simulink model "charttest"  (R2014b)
settings: Solver=ode45  StartTime=0.0  StopTime=30  RelTol=1e-3
libraries: simulink x2
settings Model: Creator=Edoardo  LastModifiedBy=Edoardo
settings SolverCC: PositivePriorityOrder=on

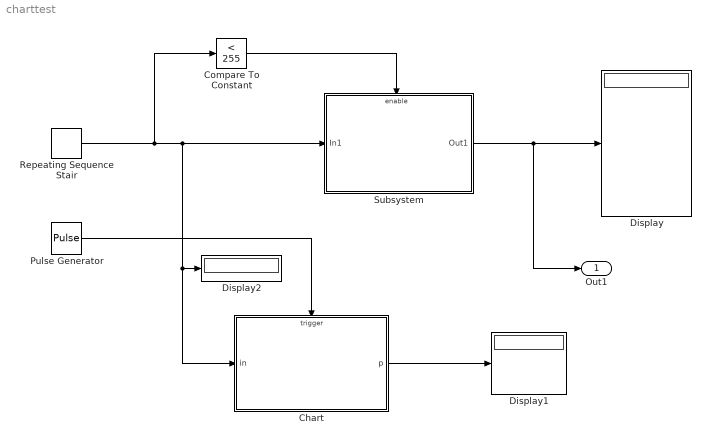
== system charttest ==
  Chart : Stateflow chart  TreatAsAtomicUnit=on
  Compare To Constant : simulink/Logic and Bit Operations/Compare To Constant  relop=<  const=255  OutDataTypeStr=boolean
  Display : Display
  Display1 : Display
  Display2 : Display
  Pulse Generator : DiscretePulseGenerator  SampleTime=0.05
  Repeating Sequence Stair : simulink/Sources/Repeating Sequence Stair  OutValues=[1 2 3 0 5 6 7 255].'  tsamp=1  OutMin=[]  OutMax=[]  OutDataTypeStr=double  OutputDataTypeScalingMode=double  OutDataType=fixdt(0,8)  ConRadixGroup=Best Precision: Vector-wise  OutScaling=2^-12
  Subsystem : Subsystem
  Out1 : Outport
  wires:
  Repeating Sequence Stair/1 -> Compare To Constant/1, Display2/1, Chart/1(in), Subsystem/1(In1)
  Compare To Constant/1 -> Subsystem/Enable
  Subsystem/1(Out1) -> Out1/1, Display/1
  Chart/1(p) -> Display1/1
  Pulse Generator/1 -> Chart/Trigger

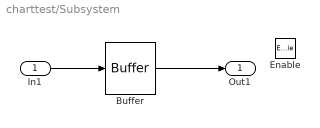
== system charttest/Subsystem ==
  In1 : Inport
  Enable : EnablePort
  Buffer : Buffer  N=4  TreatMby1Signals=One channel
  Out1 : Outport
  wires:
  In1/1 -> Buffer/1
  Buffer/1 -> Out1/1

== stateflow chart charttest/Chart ==
  state Parser
    entry:
    i = 1;
    p = 0;
    state WAITING_HEAD
    state INCOMING_DATA
      entry:
      p(i) = in;
      i = i+1;
    (default) -> WAITING_HEAD
    (junction 19) -> WAITING_HEAD [order 1] : [in == 255]
    WAITING_HEAD -> INCOMING_DATA : [in == 0]
    INCOMING_DATA -> (junction 19) : NEWDATA
    (junction 19) -> INCOMING_DATA [order 2]
  (default) -> Parser
  data: in input size=1; p output size=20; i local
  events: NEWDATA input RISING_EDGE_EVENT
